simulink model "QArm_TeleopServer"  (R2018a)
settings: Solver=ode4  StartTime=0.0  StopTime=inf  FixedStep=1/500  RelTol=1e-3  EnableMultiTasking=on
undefined symbols (not defined in the file): HIL, qc_get_step_size, Video3D
libraries: quarc_library x19, simulink x11
settings Model: SimulationMode=external  ExtModeBatchMode=on  ExtModeTrigDuration=10000  Creator=fvranes  LastModifiedBy=mrushton
settings SolverCC: PositivePriorityOrder=on
settings DataIOCC: SaveOutput=off  SignalLogging=off  DSMLogging=off  SaveTime=off
settings RTWCC: Description=QUARC Win64 Target Using Toolchain  SystemTargetFile=quarc_win64.tlc  TemplateMakefile=quarc_default_tmf  Toolchain=QUARC win64 | nmake (64-bit Windows)  BuildConfiguration=Faster Runs
settings CodeAppCC: StateflowObjectComments=on
settings STFCustomTargetCC: TargetLangStandard=C99 (ISO)  ConcurrentExecutionCompliant=on  UseToolchainInfoCompliant=on  SystemTargetFile=quarc_win64.tlc
settings GRTTargetCC: ParMdlRefBuildCompliant=off  CompOptLevelCompliant=off  CombineOutputUpdateFcns=off  MatFileLogging=off  CPPClassGenCompliant=off  GRTInterface=on  ExtMode=on  ExtModeMexFile=quarc_comm
settings ConfigComp: CovMetricSettings=dswe

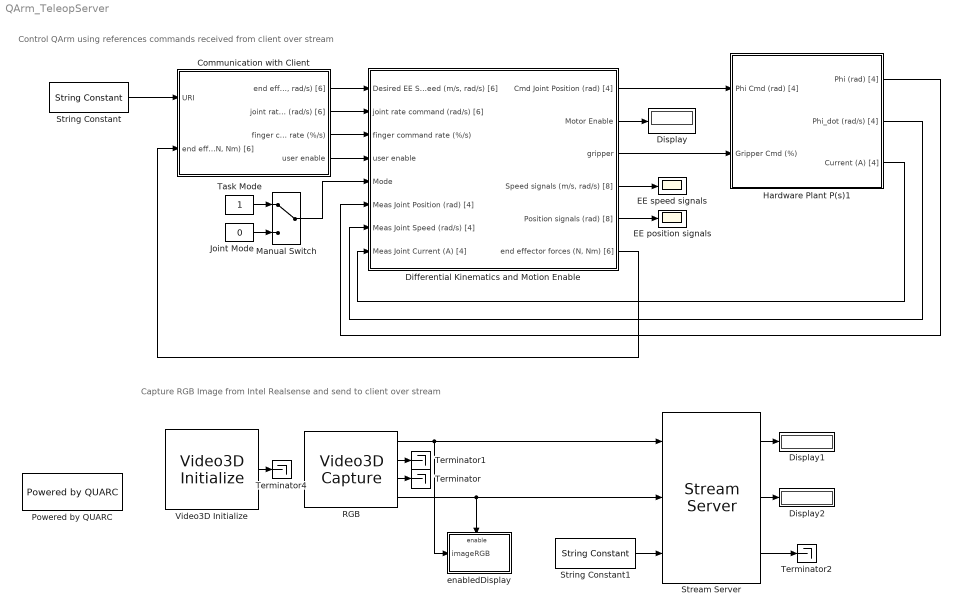
== system QArm_TeleopServer ==
  note: Control QArm using references commands received from client over stream
  note: Capture RGB Image from Intel Realsense and send to client over stream
  Communication with Client : Subsystem
  Differential Kinematics and Motion Enable : Subsystem
  Display : Display
  Display1 : Display
  Display2 : Display
  EE position signals : Scope
  EE speed signals : Scope
  Hardware Plant P(s)1 : Subsystem
  Joint Mode : Constant  Value=0
  Manual Switch : ManualSwitch
  Powered by QUARC : quarc_library/Logos/Powered by QUARC
  RGB : quarc_library/Multimedia/Video3D Capture  object_name=Video3D-1  stream_type=RGB  stream_index=0  resolution=640 x 480  width=640  height=480  output_format=MATLAB RGB (HxWx3)  data_type=uint8  sample_time=qc_get_step_size * ceil(0.033 / qc_get_step_size)  camera_intrinsics=off  depth_scale=off  brightness_override=off  brightness=50.0  contrast_override=off  contrast=50.0  hue_override=off  hue=50.0  saturation_override=off  saturation=50.0  sharpness_override=off  sharpness=50.0  gamma_override=off  gamma=50.0  gain_override=off  gain=50.0  backlightcompensation_override=off  backlightcompensation=50.0  whitebalance_override=Automatic white balance  whitebalance=50.0  exposure_override=Automatic exposure  exposure=30.0  emitter=Enable laser emitter  preset=Do not set camera presets
  Stream Server : quarc_library/Communications/Basic/Stream Server  uri_source=External input port  uri=tcpip://localhost:18025  send_buffer_size=640*480*3  receive_buffer_size=14  byte_order=little endian (Intel - LSB first)  optimization=Minimum latency  send_options=Send most recent data  receive_options=Do not receive data  default_value=zeros(14, 1)  sample_time=qc_get_step_size * ceil(0.033 / qc_get_step_size)  active=off  implementation=Use blocking I/O in a separate thread  send_fifo_size=2  receive_fifo_size=2  send_priority=0  receive_priority=0  send_dimensions=off  receive_dimensions=off  max_dimensions=-1  data_type=uint8  type_expr=BusObject
  String Constant : quarc_library/Strings/String Constant  string_value=tcpip://localhost:18018  evaluate_string=off  string_type=text  max_length=80  sample_time=inf  variable_size=off
      settings: AttributesFormatString="\"tcpip://localhost:18018\""  SourceProductName=QUARC Targets
  String Constant1 : quarc_library/Strings/String Constant  string_value=tcpip://localhost:18025  evaluate_string=off  string_type=text  max_length=80  sample_time=inf  variable_size=off
      settings: AttributesFormatString="\"tcpip://localhost:18025\""  SourceProductName=QUARC Targets
  Task Mode : Constant
  Terminator{,1..2,4} (4 alike) : Terminator
  Video3D Initialize : quarc_library/Multimedia/Video3D Initialize  object_name=Video3D-1  source=Device  identifier=0  file=sample.bag  sample_time=qc_get_step_size * ceil(0.033 / qc_get_step_size)  active=on
  enabledDisplay : Subsystem
  wires:
  Hardware Plant P(s)1/2(Phi_dot (rad/s) [4]) -> Differential Kinematics and Motion Enable/7(Meas Joint Speed (rad/s) [4])
  Differential Kinematics and Motion Enable/1(Cmd Joint Position (rad) [4]) -> Hardware Plant P(s)1/1(Phi Cmd (rad) [4])
  Hardware Plant P(s)1/1(Phi (rad) [4]) -> Differential Kinematics and Motion Enable/6(Meas Joint Position (rad) [4])
  Communication with Client/1("end effector speed (m/s, rad/s) [6]") -> Differential Kinematics and Motion Enable/1("Desired EE Speed (m/s, rad/s) [6]")
  Communication with Client/2(joint rate command (rad/s) [6]) -> Differential Kinematics and Motion Enable/2(joint rate command (rad/s) [6])
  Communication with Client/3(finger command rate (%/s)) -> Differential Kinematics and Motion Enable/3(finger command rate (%/s))
  Communication with Client/4(user enable) -> Differential Kinematics and Motion Enable/4(user enable)
  Task Mode/1 -> Manual Switch/1
  Joint Mode/1 -> Manual Switch/2
  Manual Switch/1 -> Differential Kinematics and Motion Enable/5(Mode)
  Differential Kinematics and Motion Enable/4("Speed signals (m/s, rad/s) [8]") -> EE speed signals/1
  Differential Kinematics and Motion Enable/5(Position signals (rad) [8]) -> EE position signals/1
  Differential Kinematics and Motion Enable/6("end effector forces (N, Nm) [6]") -> Communication with Client/2("end effector forces (N, Nm) [6]")
  Hardware Plant P(s)1/3(Current (A) [4]) -> Differential Kinematics and Motion Enable/8(Meas Joint Current (A) [4])
  Differential Kinematics and Motion Enable/2(Motor Enable) -> Display/1
  Differential Kinematics and Motion Enable/3(gripper) -> Hardware Plant P(s)1/2(Gripper Cmd (%))
  RGB/1 -> Stream Server/1, enabledDisplay/1(imageRGB)
  Stream Server/2 -> Display2/1
  Video3D Initialize/1 -> Terminator4/1
  RGB/4 -> Stream Server/2, enabledDisplay/Enable
  RGB/3 -> Terminator/1
  RGB/2 -> Terminator1/1
  Stream Server/1 -> Display1/1
  String Constant/1 -> Communication with Client/1(URI)
  String Constant1/1 -> Stream Server/3
  Stream Server/3 -> Terminator2/1

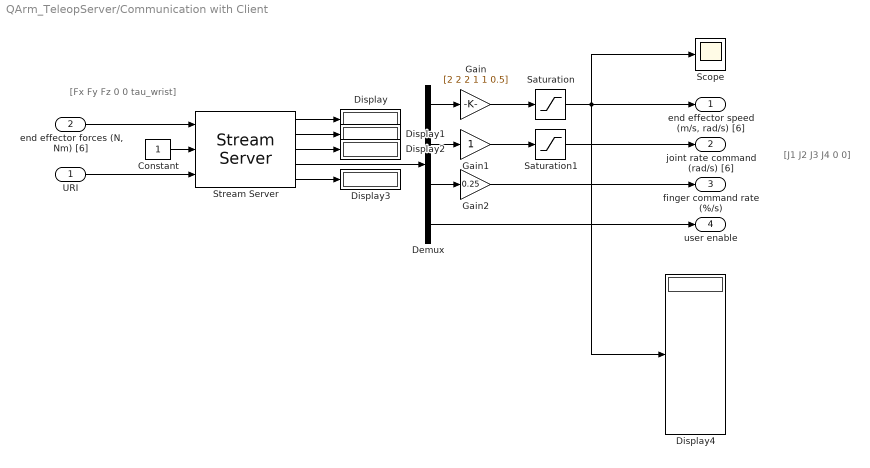
== system QArm_TeleopServer/Communication with Client ==
  note: [J1 J2 J3 J4 0 0]
  note: [Fx Fy Fz 0 0 tau_wrist]
  URI : Inport
  "end effector forces (N, Nm) [6]" : Inport  Port=2
  Constant : Constant
  Demux : Demux  Outputs=[6 6 1 1]
  Display{,1..4} (5 alike) : Display
  Gain : Gain  Gain=[2 2 2 1 1 0.5]
  Gain1 : Gain
  Gain2 : Gain  Gain=0.25
  Saturation : Saturate  UpperLimit=[0.5 0.5 0.5 1 1 1]  LowerLimit=-[0.5 0.5 0.5 1 1 1]
  Saturation1 : Saturate  UpperLimit=pi*[1 1 1 1 1 1]/6  LowerLimit=-pi*[1 1 1 1 1 1]/6
  Scope : Scope
  Stream Server : quarc_library/Communications/Basic/Stream Server  uri_source=External input port  uri=tcpip://localhost:18018  send_buffer_size=6*8*2  receive_buffer_size=14*8*2  byte_order=little endian (Intel - LSB first)  optimization=Minimum latency  send_options=Send most recent data  receive_options=Receive most recent data  default_value=zeros(14, 1)  sample_time=qc_get_step_size  active=off  implementation=Use blocking I/O in a separate thread  send_fifo_size=1000  receive_fifo_size=1000  send_priority=0  receive_priority=0  send_dimensions=off  receive_dimensions=off  max_dimensions=-1  data_type=Inherited via back propagation  type_expr=BusObject
  "end effector speed (m/s, rad/s) [6]" : Outport
  joint rate command (rad/s) [6] : Outport  Port=2
  finger command rate (%/s) : Outport  Port=3
  user enable : Outport  Port=4
  wires:
  Stream Server/3 -> Display2/1
  Constant/1 -> Stream Server/2
  Stream Server/1 -> Display/1
  Stream Server/4 -> Demux/1
  Stream Server/5 -> Display3/1
  Stream Server/2 -> Display1/1
  Demux/1 -> Gain/1
  Demux/3 -> Gain2/1
  Demux/2 -> Gain1/1
  "end effector forces (N, Nm) [6]"/1 -> Stream Server/1
  Demux/4 -> user enable/1
  Gain/1 -> Saturation/1
  Gain1/1 -> Saturation1/1
  Gain2/1 -> finger command rate (%/s)/1
  Saturation/1 -> Scope/1, Display4/1, "end effector speed (m/s, rad/s) [6]"/1
  Saturation1/1 -> joint rate command (rad/s) [6]/1
  URI/1 -> Stream Server/3

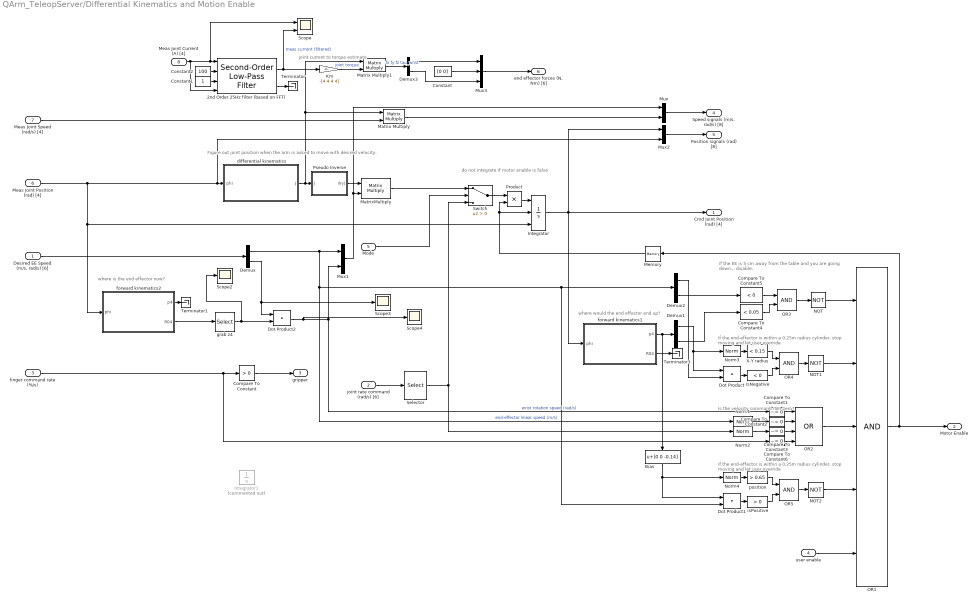
== system QArm_TeleopServer/Differential Kinematics and Motion Enable ==
  note: joint current to torque estimate
  note: do not integrate if motor enable
      | is false
  note: if the end-effector is within a 0.25m radius
      | cylinder, stop moving and let user override
  note: where would the end effector end up?
  note: if the EE is 5 cm away from the table
      | and you are going down... disable.
  note: Is the velocity command non-zero?
  note: Figure out joint position when the arm is asked to move with desired velocity.
  note: if the end-effector is within a 0.25m radius
      | cylinder, stop moving and let user override
  note: where is the end effector now?
  "Desired EE Speed (m/s, rad/s) [6]" : Inport  PortDimensions=6
  joint rate command (rad/s) [6] : Inport  Port=2
  finger command rate (%/s) : Inport  Port=3
  user enable : Inport  Port=4
  Mode : Inport  Port=5
  Meas Joint Position (rad) [4] : Inport  Port=6  PortDimensions=4
  Meas Joint Speed (rad/s) [4] : Inport  Port=7
  Meas Joint Current (A) [4] : Inport  Port=8
  2nd Order 25Hz filter (based on FFT) : quarc_library/Continuous/Second-Order Low-Pass Filter  params_source=External (input ports)  input_width=25*2*pi  input_zeta=1  input_init=0
  Bias : Bias  Bias=[0 0 -0.14]
  Compare To Constant : simulink/Logic and Bit Operations/Compare To Constant  relop=>  const=0  OutDataTypeStr=boolean
  Compare To Constant{1..3,6} (4 alike) : simulink/Logic and Bit Operations/Compare To Constant  relop=~=  const=0  OutDataTypeStr=boolean
  Compare To Constant4 : simulink/Logic and Bit Operations/Compare To Constant  relop=<  const=0.05  OutDataTypeStr=boolean
  Compare To Constant5 : simulink/Logic and Bit Operations/Compare To Constant  relop=<  const=0  OutDataTypeStr=boolean
  Constant : Constant  Value=[0 0]
  Constant1 : Constant
  Constant2 : Constant  Value=100
  Demux : Demux  Outputs=[3 3]
  Demux1 : Demux  Outputs=[2 1]
  Demux2 : Demux  Outputs=[2 1]
  Demux3 : Demux  Outputs=[3 1]
  Dot Product : DotProduct  InputSameDT=on  OutDataTypeStr=Inherit: Inherit via internal rule
  Dot Product1 : DotProduct  InputSameDT=on  OutDataTypeStr=Inherit: Inherit via internal rule
  Dot Product2 : DotProduct  InputSameDT=on  OutDataTypeStr=Inherit: Inherit via internal rule
  Integrator : Integrator  ExternalReset=falling  InitialConditionSource=external
  Integrator1 : Integrator  Commented=on  InitialCondition=0.1  LimitOutput=on  UpperSaturationLimit=0.9  LowerSaturationLimit=0.1
  IsNegative : simulink/Logic and Bit Operations/Compare To Zero  relop=<  OutDataTypeStr=boolean
  Km : Gain  Gain=-[4 4 4 4]
  Matrix Multiply : Product  Multiplication=Matrix(*)
  Matrix Multiply1 : Product  Multiplication=Matrix(*)
  MatrixMultiply : Product  Multiplication=Matrix(*)
  Memory : Memory
  Mux : Mux  Inputs=2
  Mux1 : Mux  Inputs=2
  Mux2 : Mux  Inputs=2
  Mux3 : Mux  Inputs=3
  NOT : Logic  Operator=NOT  IconShape=distinctive  AllPortsSameDT=off  OutDataTypeStr=boolean
  NOT1 : Logic  Operator=NOT  IconShape=distinctive  AllPortsSameDT=off  OutDataTypeStr=boolean
  NOT2 : Logic  Operator=NOT  IconShape=distinctive  AllPortsSameDT=off  OutDataTypeStr=boolean
  Norm{1..4} (4 alike) : quarc_library/Math Operations/Vectors/Norm
      settings: SourceProductName=QUARC Targets
  OR1 : Logic  Inputs=5  IconShape=distinctive  AllPortsSameDT=off  OutDataTypeStr=boolean
  OR2 : Logic  Operator=OR  Inputs=4  IconShape=distinctive  AllPortsSameDT=off  OutDataTypeStr=boolean
  OR3 : Logic  IconShape=distinctive  AllPortsSameDT=off  OutDataTypeStr=boolean
  OR4 : Logic  IconShape=distinctive  AllPortsSameDT=off  OutDataTypeStr=boolean
  OR5 : Logic  IconShape=distinctive  AllPortsSameDT=off  OutDataTypeStr=boolean
  Product : Product
  Pseudo Inverse : MATLAB Function  TreatAsAtomicUnit=on
  Scope : Scope  NumInputPorts=2
  Scope2 : Scope
  Scope3 : Scope
  Scope4 : Scope
  Selector : Selector  InputPortWidth=6  IndexOptions=Index vector (dialog)  Indices=[1:4]  OutputSizes=1
  Switch : Switch  Criteria=u2 > Threshold
  Terminator : Terminator
  Terminator1 : Terminator
  Terminator3 : Terminator
  X-Y radius : simulink/Logic and Bit Operations/Compare To Constant  relop=<  const=0.15  OutDataTypeStr=boolean
  differential kinematics : MATLAB Function  TreatAsAtomicUnit=on
  forward kinematics1 : MATLAB Function  TreatAsAtomicUnit=on
  forward kinematics2 : MATLAB Function  TreatAsAtomicUnit=on
  grab z4 : Selector  NumberOfDimensions=2  InputPortWidth=3  IndexOptions=Index vector (dialog),Index vector (dialog)  Indices=[1:3],3  OutputSizes=1,1
  isPositive : simulink/Logic and Bit Operations/Compare To Zero  relop=>  OutDataTypeStr=boolean
  position : simulink/Logic and Bit Operations/Compare To Constant  relop=>  const=0.65  OutDataTypeStr=boolean
  Cmd Joint Position (rad) [4] : Outport  VectorParamsAs1DForOutWhenUnconnected=off
  Motor Enable : Outport  Port=2  VectorParamsAs1DForOutWhenUnconnected=off
  gripper : Outport  Port=3
  "Speed signals (m/s, rad/s) [8]" : Outport  Port=4
  Position signals (rad) [8] : Outport  Port=5
  "end effector forces (N, Nm) [6]" : Outport  Port=6
  wires:
  Compare To Constant2/1 -> OR2/2
  Demux/1 -> Dot Product1/2, Demux2/1, Norm1/1, Mux1/1  "end-effector linear speed (m/s)"
  OR1/1 -> Memory/1, Motor Enable/1
  Meas Joint Position (rad) [4]/1 -> Mux2/2, differential kinematics/1(phi), Integrator/3, forward kinematics2/1(phi)
  Integrator/1 -> Mux2/1, Cmd Joint Position (rad) [4]/1, forward kinematics1/1(phi)
  Compare To Constant4/1 -> OR3/2
  forward kinematics1/2(R04) -> Terminator3/1
  Pseudo Inverse/1(invJ) -> MatrixMultiply/1
  MatrixMultiply/1 -> Switch/1
  Norm1/1 -> Compare To Constant2/1
  Dot Product2/1 -> Scope4/1, Mux1/2, Compare To Constant1/1  "wrist rotation speed (rad/s)"
  Demux1/2 -> Compare To Constant4/1
  Mux1/1 -> Mux/1, MatrixMultiply/2
  "Desired EE Speed (m/s, rad/s) [6]"/1 -> Demux/1
  Demux/2 -> Scope3/1, Dot Product2/1
  Compare To Constant1/1 -> OR2/1
  OR2/1 -> OR1/3
  Demux2/2 -> Compare To Constant5/1
  Compare To Constant5/1 -> OR3/1
  OR3/1 -> NOT/1
  NOT/1 -> OR1/1
  Memory/1 -> Product/2, Integrator/2
  Product/1 -> Integrator/1
  Demux2/1 -> Dot Product/2
  Demux1/1 -> Dot Product/1, Norm3/1
  Norm3/1 -> X-Y radius/1
  X-Y radius/1 -> OR4/1
  NOT1/1 -> OR1/2
  OR4/1 -> NOT1/1
  Dot Product/1 -> IsNegative/1
  IsNegative/1 -> OR4/2
  Meas Joint Speed (rad/s) [4]/1 -> Matrix Multiply/2
  Matrix Multiply/1 -> Mux/2
  Mux/1 -> "Speed signals (m/s, rad/s) [8]"/1
  Mux2/1 -> Position signals (rad) [8]/1
  joint rate command (rad/s) [6]/1 -> Selector/1
  Mode/1 -> Switch/2
  Switch/1 -> Product/1
  Selector/1 -> Norm2/1, Switch/3
  Meas Joint Current (A) [4]/1 -> Scope/1, 2nd Order 25Hz filter (based on FFT)/1, 2nd Order 25Hz filter (based on FFT)/4
  differential kinematics/1(J) -> Matrix Multiply1/1, Matrix Multiply/1, Pseudo Inverse/1(J)
  Km/1 -> Matrix Multiply1/2  "joint torque"
  Matrix Multiply1/1 -> Demux3/1  "fx fy fz tau_wrist"
  Demux3/1 -> Mux3/1
  Demux3/2 -> Mux3/3
  Constant/1 -> Mux3/2
  Mux3/1 -> "end effector forces (N, Nm) [6]"/1
  2nd Order 25Hz filter (based on FFT)/1 -> Scope/2, Km/1  "meas current (filtered)"
  2nd Order 25Hz filter (based on FFT)/2 -> Terminator/1
  Constant1/1 -> 2nd Order 25Hz filter (based on FFT)/3
  Constant2/1 -> 2nd Order 25Hz filter (based on FFT)/2
  Norm2/1 -> Compare To Constant3/1
  Compare To Constant3/1 -> OR2/3
  Compare To Constant6/1 -> OR2/4
  finger command rate (%/s)/1 -> Compare To Constant/1, Compare To Constant6/1
  Norm4/1 -> position/1
  OR5/1 -> NOT2/1
  isPositive/1 -> OR5/2
  Dot Product1/1 -> isPositive/1
  position/1 -> OR5/1
  NOT2/1 -> OR1/4
  user enable/1 -> OR1/5
  forward kinematics1/1(p4) -> Demux1/1, Bias/1
  Bias/1 -> Norm4/1, Dot Product1/1
  Compare To Constant/1 -> gripper/1
  forward kinematics2/1(p4) -> Terminator1/1
  forward kinematics2/2(R04) -> grab z4/1
  grab z4/1 -> Scope2/1, Dot Product2/2

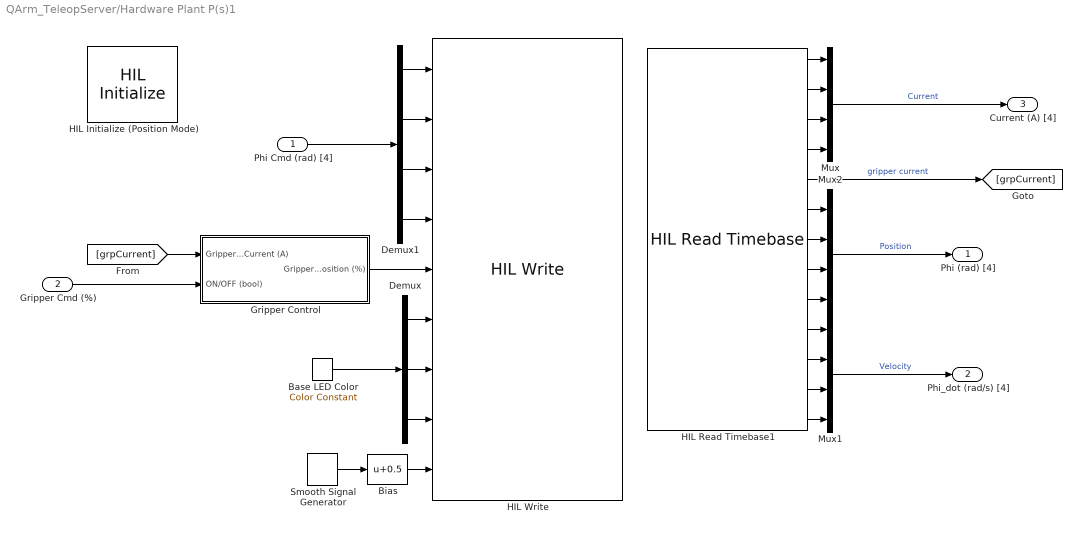
== system QArm_TeleopServer/Hardware Plant P(s)1 ==
  Phi Cmd (rad) [4] : Inport
  Gripper Cmd (%) : Inport  Port=2
  Base LED Color : quarc_library/Sources/Signals/Color Constant  color=[0 1 0]
      settings: SourceProductName=QUARC Targets
  Bias : Bias  Bias=0.5
  Demux : Demux  Outputs=3
  Demux1 : Demux
  Gripper Control : Subsystem
  HIL Initialize (Position Mode) : quarc_library/Data Acquisition/Generic/Configuration/HIL Initialize  object_name=HIL-1  board_type=qarm_usb  board_number=0  board_options=j0_mode=0;j1_mode=0;j2_mode=0;j3_mode=0;gripper_mode=0;j0_profile_config=0;j0_profile_velocity=0;j0_profile_acceleration=0;j1_profile_config=0;j1_profile_velocity=0;j1_profile_acceleration=0;j2_profile_config=0;j2_profile_velocity=0;j2_profile_acceleration=0;j3_profile_config=0;j3_profile_velocity=0;j3_profile_acceleration=0;  exclusive=off  active=on  hardware_clocks=[0]  clock_modes=[]  initial_clock_frequencies=[]  set_clock_params_at_start=off  set_clock_params_at_switch_in=off  set_clock_frequencies_at_start=off  set_clock_frequencies_at_switch_in=off  analog_input_channels=[5:9]  analog_input_configurations=[]  analog_input_maximums=[]  analog_input_minimums=[]  set_analog_input_params_at_start=off  set_analog_input_params_at_switch_in=off  analog_output_channels=[]  analog_output_maximums=inf  analog_output_minimums=-inf  initial_analog_outputs=[0]  final_analog_outputs=[0]  watchdog_analog_outputs=[]  set_analog_output_params_at_start=off  set_analog_output_params_at_switch_in=off  set_analog_outputs_at_start=off  set_analog_outputs_at_switch_in=off  set_analog_outputs_at_terminate=off  set_analog_outputs_at_switch_out=off  set_analog_outputs_on_watchdog=off  digital_input_channels=[]  digital_output_channels=[]  digital_output_configuration=[]  initial_digital_outputs=[0]  final_digital_outputs=[0]  watchdog_digital_outputs=[0]  set_digital_output_params_at_start=off  set_digital_output_params_at_switch_in=off  set_digital_outputs_at_start=off  set_digital_outputs_at_switch_in=off  set_digital_outputs_at_terminate=off  set_digital_outputs_at_switch_out=off  set_digital_outputs_on_watchdog=off  encoder_channels=[]  quadrature=[]  encoder_filter_frequency=[]  initial_encoder_counts=[]  set_encoder_params_at_start=off  set_encoder_params_at_switch_in=off  set_encoder_counts_at_start=off  set_encoder_counts_at_switch_in=off  pwm_channels=[]  pwm_modes=[]  pwm_frequency=[]  pwm_configuration=[]  pwm_alignment=[]  pwm_polarity=[]  pwm_leading_deadband=[]  pwm_trailing_deadband=[]  initial_pwm_outputs=[]  final_pwm_outputs=[]  watchdog_pwm_outputs=[]  set_pwm_params_at_start=off  set_pwm_params_at_switch_in=off  set_pwm_outputs_at_start=off  set_pwm_outputs_at_switch_in=off  set_pwm_outputs_at_terminate=off  set_pwm_outputs_at_switch_out=off  set_pwm_outputs_on_watchdog=off  other_output_channels=[11005:11008 1000:1004 11000:11003]  initial_other_outputs=[zeros(1,9), ones(1,3)]  final_other_outputs=[1 0 0 0]  watchdog_other_outputs=zeros(1,12)  set_other_outputs_at_start=off  set_other_outputs_at_switch_in=off  set_other_outputs_at_terminate=on  set_other_outputs_at_switch_out=off  set_other_outputs_on_watchdog=off
  HIL Read Timebase1 : quarc_library/Data Acquisition/Generic/Timebases/HIL Read Timebase  object_name=HIL-1  clock=0  analog_channels=[5:9]  encoder_channels=[]  digital_channels=[]  other_channels=[1000:1003 3000:3003]  active=on  vector_output=off  data_type_mode=Inherit via back propagation  encoder_data_type=double  digital_data_type=boolean  overflow_mode=Error on overflow  samples_in_buffer=max(ceil(1/qc_get_step_size), 1)
  HIL Write : quarc_library/Data Acquisition/Generic/Immediate I//O/HIL Write  object_name=HIL-1  analog_channels=[]  pwm_channels=[]  digital_channels=[]  other_channels=[1000:1004 11005:11008]  sample_time=-1  active=on  vector_input=off
  Mux : Mux
  Mux1 : Mux
  Mux2 : Mux
  Smooth Signal Generator : quarc_library/Sources/Signals/Smooth Signal Generator  signal_type=Sine  source=Internal (dialog parameters)  amplitude=0.5  frequency=0.5  initial_phase=0  sample_time=qc_get_step_size  output_cos=off
      settings: SourceProductName=QUARC Targets
  Phi (rad) [4] : Outport  VectorParamsAs1DForOutWhenUnconnected=off
  Phi_dot (rad/s) [4] : Outport  Port=2  VectorParamsAs1DForOutWhenUnconnected=off
  Current (A) [4] : Outport  Port=3  VectorParamsAs1DForOutWhenUnconnected=off
  wires:
  Gripper Cmd (%)/1 -> Gripper Control/2(ON/OFF (bool))
  Mux2/1 -> Phi (rad) [4]/1  "Position"
  Phi Cmd (rad) [4]/1 -> Demux1/1
  Demux1/4 -> HIL Write/4
  Demux1/3 -> HIL Write/3
  Demux1/2 -> HIL Write/2
  Demux1/1 -> HIL Write/1
  Base LED Color/1 -> Demux/1
  Mux1/1 -> Phi_dot (rad/s) [4]/1  "Velocity"
  Mux/1 -> Current (A) [4]/1  "Current"
  HIL Read Timebase1/1 -> Mux/1
  HIL Read Timebase1/2 -> Mux/2
  Demux/2 -> HIL Write/7
  Demux/1 -> HIL Write/6
  HIL Read Timebase1/3 -> Mux/3
  Demux/3 -> HIL Write/8
  HIL Read Timebase1/5 -> [grpCurrent]  "gripper current"
  HIL Read Timebase1/7 -> Mux2/2
  HIL Read Timebase1/4 -> Mux/4
  HIL Read Timebase1/8 -> Mux2/3
  HIL Read Timebase1/6 -> Mux2/1
  HIL Read Timebase1/9 -> Mux2/4
  Smooth Signal Generator/1 -> Bias/1
  Bias/1 -> HIL Write/9
  Gripper Control/1(Gripper Position (%)) -> HIL Write/5
  [grpCurrent] -> Gripper Control/1(Gripper Current (A))
  HIL Read Timebase1/10 -> Mux1/1
  HIL Read Timebase1/11 -> Mux1/2
  HIL Read Timebase1/12 -> Mux1/3
  HIL Read Timebase1/13 -> Mux1/4

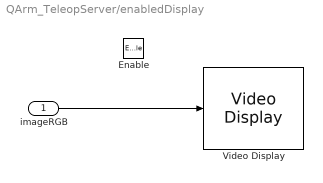
== system QArm_TeleopServer/enabledDisplay ==
  imageRGB : Inport
  Enable : EnablePort  PropagateVarSize=During execution
  Video Display : quarc_library/Multimedia/Video Display  Tag=QArm_TeleopServer/enabledDisplay/Video Display  sample_time=-1  use_hardware=on
  wires:
  imageRGB/1 -> Video Display/1

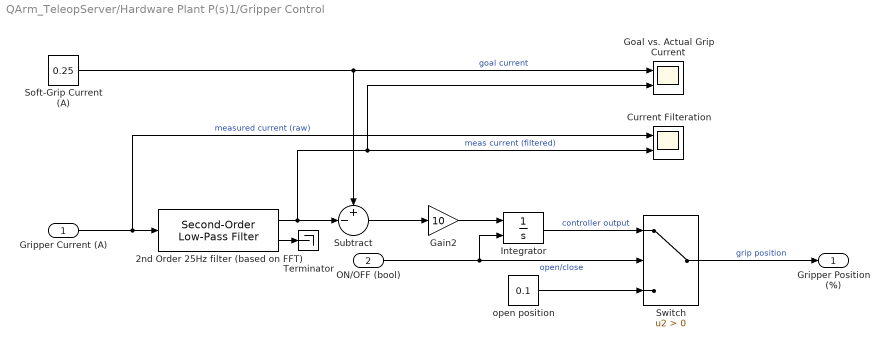
== system QArm_TeleopServer/Hardware Plant P(s)1/Gripper Control ==
  Gripper Current (A) : Inport
  ON/OFF (bool) : Inport  Port=2
  2nd Order 25Hz filter (based on FFT) : quarc_library/Continuous/Second-Order Low-Pass Filter  params_source=Internal (dialog parameters)  input_width=25*2*pi  input_zeta=1  input_init=0
  Current Filteration : Scope  NumInputPorts=2
  Gain2 : Gain  Gain=10
  Goal vs. Actual Grip Current : Scope  NumInputPorts=2
  Integrator : Integrator  ExternalReset=either  InitialCondition=0.1  LimitOutput=on  UpperSaturationLimit=0.9  LowerSaturationLimit=0.1
  Soft-Grip Current (A) : Constant  Value=0.25
  Subtract : Sum  Inputs=+-|
  Switch : Switch  Criteria=u2 > Threshold
  Terminator : Terminator
  open position : Constant  Value=0.1
  Gripper Position (%) : Outport  VectorParamsAs1DForOutWhenUnconnected=off
  wires:
  Gripper Current (A)/1 -> 2nd Order 25Hz filter (based on FFT)/1, Current Filteration/1  "measured current (raw)"
  ON/OFF (bool)/1 -> Switch/2, Integrator/2  "open/close"
  open position/1 -> Switch/3
  Switch/1 -> Gripper Position (%)/1  "grip position"
  Soft-Grip Current (A)/1 -> Subtract/1, Goal vs. Actual Grip Current/1  "goal current"
  2nd Order 25Hz filter (based on FFT)/1 -> Subtract/2, Current Filteration/2, Goal vs. Actual Grip Current/2  "meas current (filtered)"
  Subtract/1 -> Gain2/1
  Integrator/1 -> Switch/1  "controller output"
  Gain2/1 -> Integrator/1
  2nd Order 25Hz filter (based on FFT)/2 -> Terminator/1

== matlab function QArm_TeleopServer/Differential Kinematics and Motion Enable/forward kinematics2 ==
  data: phi input; p4 output; R04 output
function [p4, R04] = qarmForwardKinematics(phi)

%% QUANSER_ARM_FPK
% v 4.0 - 4th June 2020

% REFERENCE: 
% Chapter 3. Forward Kinematics
% Robot Dynamics and Control 
% Spong, Vidyasagar
% 1989

% INPUTS:
% phi     : Alternate joint angles vector 4 x 1

% OUTPUTS:
% p4      : End-effector frame {4} position vector expressed in base frame {0}
% R04     : rotation matrix from end-effector frame {4} to base frame {0}

%% Manipulator parameters:
L1 = 0.1400;
L2 = 0.3500;
L3 = 0.0500;
L4 = 0.2500;
L5 = 0.1500;

%% Alternate parameters
l1 = L1;
l2 = sqrt(L2^2 + L3^2);
l3 = L4 + L5;
beta = atan(L3/L2);

%% From phi space to theta space 
theta = phi;
theta(1) = phi(1);
theta(2) = phi(2) + beta - pi/2;
theta(3) = phi(3) - beta;
theta(4) = phi(4);

%% Transformation matrices for all frames:

% T{i-1}{i} = quanser_arm_DH(  a, alpha,  d,     theta );
        T01 = quanser_arm_DH(  0, -pi/2, l1,  theta(1) );
        T12 = quanser_arm_DH( l2,     0,  0,  theta(2) );
        T23 = quanser_arm_DH(  0, -pi/2,  0,  theta(3) );
        T34 = quanser_arm_DH(  0,     0, l3,  theta(4) );

        T02 = T01*T12;
        T03 = T02*T23;
        T04 = T03*T34;

%% Position of end-effector Transformation

% Extract the Position vector 
% p1   = T01(1:3,4);
% p2   = T02(1:3,4);
% p3   = T03(1:3,4);
p4   = T04(1:3,4);

% Extract the Rotation matrix
% R01 = T01(1:3,1:3);
% R02 = T02(1:3,1:3);
% R03 = T03(1:3,1:3);
R04 = T04(1:3,1:3);

end

function T = quanser_arm_DH(a,alpha,d,theta)

%% QUANSER_ARM_DH
% v 1.0 - 26th March 2019

% REFERENCE: 
% Chapter 3. Forward and Inverse Kinematics
% Robot Modeling and Control 
% Spong, Hutchinson, Vidyasagar
% 2006

% INPUTS:
% a       :   translation  : along : x_{i}   : from : z_{i-1} : to : z_{i}
% alpha   :      rotation  : about : x_{i}   : from : z_{i-1} : to : z_{i}
% d       :   translation  : along : z_{i-1} : from : x_{i-1} : to : x_{i}
% theta   :      rotation  : about : z_{i-1} : from : x_{i-1} : to : x_{i}
% NOTE: Standard DH Parameters

% OUTPUTS:
% T       : transformation                   : from :     {i} : to : {i-1}

%%
% Rotation Transformation about z axis by theta
T_R_z = [cos(theta) -sin(theta) 0 0;
         sin(theta)  cos(theta) 0 0;
                  0           0 1 0;
                  0           0 0 1];
     
% Translation Transformation along z axis by d
T_T_z = [1 0 0 0;
         0 1 0 0;
         0 0 1 d;
         0 0 0 1];

% Translation Transformation along x axis by a
T_T_x = [1 0 0 a;
         0 1 0 0;
         0 0 1 0;
         0 0 0 1];

% Rotation Transformation about x axis by alpha
T_R_x = [1          0           0 0;
         0 cos(alpha) -sin(alpha) 0;
         0 sin(alpha)  cos(alpha) 0;
         0          0           0 1];

% For a transformation FROM frame {i} TO frame {i-1}: A
T = T_R_z*T_T_z*T_T_x*T_R_x;

end

== matlab function QArm_TeleopServer/Differential Kinematics and Motion Enable/differential kinematics ==
  data: phi input; J output
function J   = qarmDifferentialKinematics(phi)

%% QUANSER_ARM_FDK
% v 1.0 - 13th August 2020

% REFERENCE: 
% Chapter 5. Velocity Kinematics
% Robot Dynamics and Control 
% Spong, Vidyasagar
% 1989

% INPUTS:
% phi     : Alternate joint angles vector 4 x 1

% OUTPUTS:
% p4      : End-effector frame {4} position vector expressed in base frame {0}
% R04     : rotation matrix from end-effector frame {4} to base frame {0}

%% Manipulator parameters:
L1 = 0.1400;
L2 = 0.3500;
L3 = 0.0500;
L4 = 0.2500;
L5 = 0.1500;

%% Alternate parameters
l1 = L1;
l2 = sqrt(L2^2 + L3^2);
l3 = L4 + L5;
beta = atan(L3/L2);

%% From phi space to theta space 
theta = phi;
theta(1) = phi(1);
theta(2) = phi(2) + beta - pi/2;
theta(3) = phi(3) - beta;
theta(4) = phi(4);

%% Jacobian term definition:

J = eye(4);
J(1,1) = - l2*sin(theta(1))*cos(theta(2)) + l3*sin(theta(1))*sin(theta(2)+theta(3)); 
J(1,2) = - l2*cos(theta(1))*sin(theta(2)) - l3*cos(theta(1))*cos(theta(2)+theta(3)); 
J(1,3) = - l3*cos(theta(1))*cos(theta(2)+theta(3)); 
J(1,4) = 0;
J(2,1) =   l2*cos(theta(1))*cos(theta(2)) - l3*cos(theta(1))*sin(theta(2)+theta(3)); 
J(2,2) = - l2*sin(theta(1))*sin(theta(2)) - l3*sin(theta(1))*cos(theta(2)+theta(3)); 
J(2,3) = - l3*sin(theta(1))*cos(theta(2)+theta(3));
J(2,4) = 0;
J(3,1) = 0; 
J(3,2) = - l2*cos(theta(2)) + l3*sin(theta(2)+theta(3)); 
J(3,3) =   l3*sin(theta(2)+theta(3));
J(3,4) = 0;
J(4,1) = 0;
J(4,2) = 0;
J(4,3) = 0;
J(4,4) = 1;

end

== matlab function QArm_TeleopServer/Differential Kinematics and Motion Enable/forward kinematics1 ==
  data: phi input; p4 output; R04 output
function [p4, R04] = qarmForwardKinematics(phi)

%% QUANSER_ARM_FPK
% v 4.0 - 4th June 2020

% REFERENCE: 
% Chapter 3. Forward Kinematics
% Robot Dynamics and Control 
% Spong, Vidyasagar
% 1989

% INPUTS:
% phi     : Alternate joint angles vector 4 x 1

% OUTPUTS:
% p4      : End-effector frame {4} position vector expressed in base frame {0}
% R04     : rotation matrix from end-effector frame {4} to base frame {0}

%% Manipulator parameters:
L1 = 0.1400;
L2 = 0.3500;
L3 = 0.0500;
L4 = 0.2500;
L5 = 0.1500;

%% Alternate parameters
l1 = L1;
l2 = sqrt(L2^2 + L3^2);
l3 = L4 + L5;
beta = atan(L3/L2);

%% From phi space to theta space 
theta = phi;
theta(1) = phi(1);
theta(2) = phi(2) + beta - pi/2;
theta(3) = phi(3) - beta;
theta(4) = phi(4);

%% Transformation matrices for all frames:

% T{i-1}{i} = quanser_arm_DH(  a, alpha,  d,     theta );
        T01 = quanser_arm_DH(  0, -pi/2, l1,  theta(1) );
        T12 = quanser_arm_DH( l2,     0,  0,  theta(2) );
        T23 = quanser_arm_DH(  0, -pi/2,  0,  theta(3) );
        T34 = quanser_arm_DH(  0,     0, l3,  theta(4) );

        T02 = T01*T12;
        T03 = T02*T23;
        T04 = T03*T34;

%% Position of end-effector Transformation

% Extract the Position vector 
% p1   = T01(1:3,4);
% p2   = T02(1:3,4);
% p3   = T03(1:3,4);
p4   = T04(1:3,4);

% Extract the Rotation matrix
% R01 = T01(1:3,1:3);
% R02 = T02(1:3,1:3);
% R03 = T03(1:3,1:3);
R04 = T04(1:3,1:3);

end

function T = quanser_arm_DH(a,alpha,d,theta)

%% QUANSER_ARM_DH
% v 1.0 - 26th March 2019

% REFERENCE: 
% Chapter 3. Forward and Inverse Kinematics
% Robot Modeling and Control 
% Spong, Hutchinson, Vidyasagar
% 2006

% INPUTS:
% a       :   translation  : along : x_{i}   : from : z_{i-1} : to : z_{i}
% alpha   :      rotation  : about : x_{i}   : from : z_{i-1} : to : z_{i}
% d       :   translation  : along : z_{i-1} : from : x_{i-1} : to : x_{i}
% theta   :      rotation  : about : z_{i-1} : from : x_{i-1} : to : x_{i}
% NOTE: Standard DH Parameters

% OUTPUTS:
% T       : transformation                   : from :     {i} : to : {i-1}

%%
% Rotation Transformation about z axis by theta
T_R_z = [cos(theta) -sin(theta) 0 0;
         sin(theta)  cos(theta) 0 0;
                  0           0 1 0;
                  0           0 0 1];
     
% Translation Transformation along z axis by d
T_T_z = [1 0 0 0;
         0 1 0 0;
         0 0 1 d;
         0 0 0 1];

% Translation Transformation along x axis by a
T_T_x = [1 0 0 a;
         0 1 0 0;
         0 0 1 0;
         0 0 0 1];

% Rotation Transformation about x axis by alpha
T_R_x = [1          0           0 0;
         0 cos(alpha) -sin(alpha) 0;
         0 sin(alpha)  cos(alpha) 0;
         0          0           0 1];

% For a transformation FROM frame {i} TO frame {i-1}: A
T = T_R_z*T_T_z*T_T_x*T_R_x;

end

== matlab function QArm_TeleopServer/Differential Kinematics and Motion Enable/Pseudo Inverse ==
  data: J input; invJ output
function invJ = fcn(J)
invJ = pinv(J);
